simulink model "MotorControl_0"  (Simulink 8.1)
settings: Solver=FixedStepDiscrete  StartTime=0.0  StopTime=10.0  FixedStep=0.02  RelTol=1e-3
PostLoadFcn:
  | MotorControl_0_data
undefined symbols (not defined in the file or in its folder): A14, B, B13, D, L3, R10
libraries: BAMLIB564xL x8, rappid_564xl_ec_toolbox x1
CloseFcn:
  | rtwprivate ssgencode ModelCloseRequest MotorControl_1
settings Model: Creator=evarshavskaya  LastModifiedBy=evarshavskaya
settings DataIOCC: ExternalInput=off  InitialState=off  SaveOutput=off  SignalLogging=off  SaveTime=off
settings OptimizationCC: InlineParams=on  OptimizeModelRefInitCode=on  LifeSpan=1
settings DebuggingCC: InheritedTsInSrcMsg=none  SingleTaskRateTransMsg=error  ParameterPrecisionLossMsg=none  UnconnectedInputMsg=error  UnconnectedOutputMsg=error  UnconnectedLineMsg=error  UnknownTsInhSupMsg=error
settings HardwareCC: ProdLargestAtomicInteger=Long  ProdLargestAtomicFloat=Double  ProdIntDivRoundTo=Zero  ProdEndianess=BigEndian  ProdHWDeviceType=Freescale->32-bit PowerPC
settings RTWCC: SystemTargetFile=rappid564xl.tlc  MakeCommand=rappid_564xl_make_rtw  TemplateMakefile=rappid_564xl_default_tmf  PostCodeGenCommand=rappid_analyzegencode(buildInfo)  Description=RAppID Toolbox MPC564xL Code Generation Target (rappid)  ProcessScript=rappid564xl_make_rtw_hook
settings CodeAppCC: IgnoreCustomStorageClasses=off  CustomSymbolStrType=$N$R$M  InternalIdentifier=Classic
settings STFCustomTargetCC: CodeReplacementLibrary=ANSI_C  ModelReferenceCompliant=off  CombineOutputUpdateFcns=on  SuppressErrorStatus=on  ERTCustomFileBanners=on  SupportContinuousTime=off  SupportNonInlinedSFcns=off  MATLABClassNameForMDSCustomization=Simulink.SoftwareTarget.ERTCustomization  GRTInterface=off  SystemTargetFile=rappid564xl.tlc
settings ERTTargetCC: CodeReplacementLibrary=ANSI_C  MultiwordLength=2048  ModelReferenceCompliant=off  ParMdlRefBuildCompliant=off  CompOptLevelCompliant=off  ConcurrentExecutionCompliant=off  SuppressErrorStatus=on  ERTFirstTimeCompliant=off  ModelStepFunctionPrototypeControlCompliant=off  CPPClassGenCompliant=off  ExtModeMexFile=noextcomm  InlinedParameterPlacement=NonHierarchical  ERTCustomFileTemplate=example_file_process.tlc  ConvertIfToSwitch=off  SuppressUnreachableDefaultCases=off

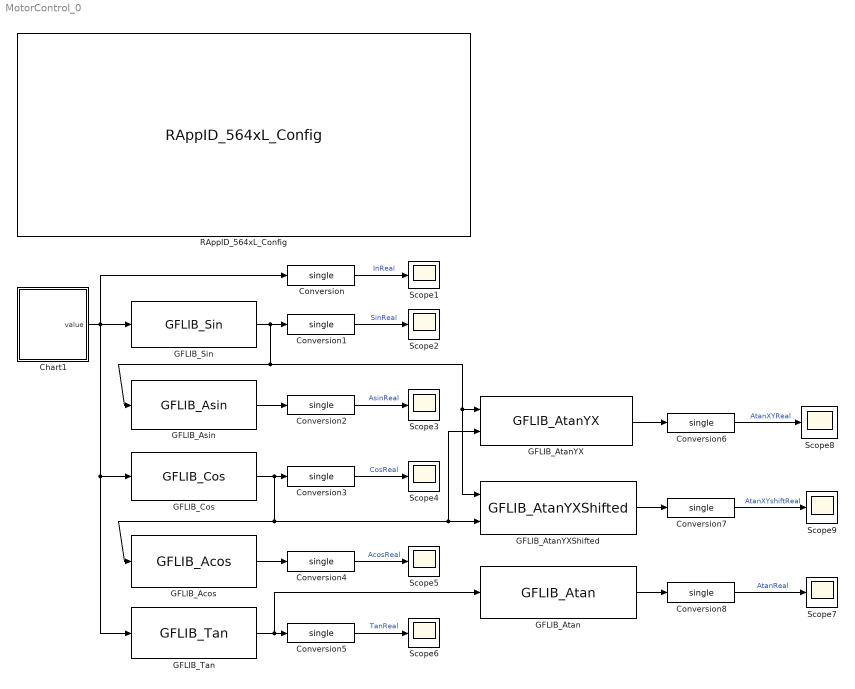
== system MotorControl_0 ==
  Chart1 : Stateflow chart  TreatAsAtomicUnit=on
  Conversion{,1..8} (9 alike) : DataTypeConversion  OutDataTypeStr=single
  GFLIB_Acos : BAMLIB564xL/General Functions/GFLIB_Acos
  GFLIB_Asin : BAMLIB564xL/General Functions/GFLIB_Asin
  GFLIB_Atan : BAMLIB564xL/General Functions/GFLIB_Atan
  GFLIB_AtanYX : BAMLIB564xL/General Functions/GFLIB_AtanYX
  GFLIB_AtanYXShifted : BAMLIB564xL/General Functions/GFLIB_AtanYXShifted  Ky=Ky  Kx=Kx  ThetaAdj=ThetaAdj
  GFLIB_Cos : BAMLIB564xL/General Functions/GFLIB_Cos
  GFLIB_Sin : BAMLIB564xL/General Functions/GFLIB_Sin
  GFLIB_Tan : BAMLIB564xL/General Functions/GFLIB_Tan
  RAppID_564xL_Config : rappid_564xl_ec_toolbox/MPC564xL/RAppID_564xL_Config  SystemClock=120  XTAL=40  MC_clock_60=12  MC_clock_80=16  MC_clock_120=10  SWG_clock_60=20  SWG_clock_80=13.334  SWG_clock_120=20  Compiler=CodeWarrior  MemTarget=RAM  Part=MPC5643L  Package=144 LQFP  global_int_priority=10  base_tick_priority=14  sys_task_supress=off  exception_handlers=off  stored_mdl_name=MotorControl_1  freemaster_interface=Oops  freemaster_rx_pin="LINFlex_0 Rx Pin 116 : \"PB[3]\""  freemaster_tx_pin="LINFlex_0 Tx Pin 114 : \"PB[2]\""  freemaster_interface_1=Serial 0  freemaster_enable=on  freemaster_rate=57600  freemaster_tx0_pin=18 : B[2] : 114 : A14  freemaster_rx0_pin=19 : B[3] : 116 : B13  freemaster_tx1_pin=57 : D[9] : 26 : L3  freemaster_rx1_pin=29 : B[13] : 60 : R10  freemaster_can_channel=1CH  freemater_can_speed=500K  freemaster_can_msgig=0x7AA  ccp_interface=None  ccp_enable=off  ccp_can_channel=CH1 (MB 0 - 1)  ccp_can_speed=500K  ccp_can_cro_id=256  ccp_can_dto_id=257  ccp_dev_id=RappID  ccp_dev_addr=0  ccp_odt=3  ccp_daq=3  pil_enable=off  pil_bam=on  comport=1  pil_rate=57600  bam_password_def=on  bam_password=0xFEEDFACECAFEBEEF  bam_sa_cs=off  bam_start_address=0x0  bam_code_size=0x7000  cons_dspi=on  cons_can=on  cons_adc=on  cons_pwm=on  cons_ctu=on  cons_swg=on  cons_eTimer=on  cons_fm=on
  Scope{1..9} (9 alike) : Scope
      Scope1 settings: TickLabels=on  TimeRange=10  YMin=-3.14  YMax=3.14
      Scope2 settings: TickLabels=on  TimeRange=10  YMin=-1  YMax=1
      Scope3 settings: TickLabels=on  TimeRange=10  YMin=-1.57  YMax=1.57  SaveName=ScopeData2
      Scope4 settings: TickLabels=on  TimeRange=10  YMin=-1  YMax=1  SaveName=ScopeData3
      Scope5 settings: TickLabels=on  TimeRange=10  YMin=0  YMax=3.14  SaveName=ScopeData4
      Scope6 settings: TickLabels=on  TimeRange=10  YMin=-140  YMax=140  SaveName=ScopeData5
      Scope7 settings: TickLabels=on  TimeRange=10  YMin=-1.57  YMax=1.57  SaveName=ScopeData6
      Scope8 settings: TickLabels=on  TimeRange=10  YMin=-3.14  YMax=3.14  SaveName=ScopeData7
      Scope9 settings: TickLabels=on  TimeRange=10  YMin=-3.14  YMax=3.14  SaveName=ScopeData8
  wires:
  GFLIB_Sin/1 -> GFLIB_Asin/1, GFLIB_AtanYX/1, GFLIB_AtanYXShifted/1, Conversion1/1
  GFLIB_Cos/1 -> GFLIB_Acos/1, GFLIB_AtanYX/2, GFLIB_AtanYXShifted/2, Conversion3/1
  GFLIB_Acos/1 -> Conversion4/1
  GFLIB_Tan/1 -> GFLIB_Atan/1, Conversion5/1
  GFLIB_Atan/1 -> Conversion8/1
  GFLIB_AtanYX/1 -> Conversion6/1
  Chart1/1(value) -> GFLIB_Sin/1, GFLIB_Cos/1, GFLIB_Tan/1, Conversion/1
  GFLIB_Asin/1 -> Conversion2/1
  GFLIB_AtanYXShifted/1 -> Conversion7/1
  Conversion/1 -> Scope1/1  "InReal"
  Conversion1/1 -> Scope2/1  "SinReal"
  Conversion2/1 -> Scope3/1  "AsinReal"
  Conversion3/1 -> Scope4/1  "CosReal"
  Conversion4/1 -> Scope5/1  "AcosReal"
  Conversion5/1 -> Scope6/1  "TanReal"
  Conversion6/1 -> Scope8/1  "AtanXYReal"
  Conversion7/1 -> Scope9/1  "AtanXYshiftReal"
  Conversion8/1 -> Scope7/1  "AtanReal"

== stateflow chart Chart1 ==
  settings: executeAtInitialization=1
  state A
    du:
    cntr=cntr+0.02;
    value=cntr;
    ex:
    cntr = -3.14;
  (default) -> A : {cntr=0;}
  A -> A : [cntr >= 3.14]
  data: cntr local single [-4..4] =0; value output single [-4..4]
